simulink model "gps_casestudy_1_4"  (R2023a)
settings: Solver=VariableStepAuto  StartTime=0.0  StopTime=10.0  RelTol=1e-3
settings Model: PacingRate=0.890000  ExtModeTrigDuration=100  Creator=simon  LastModifiedBy=simon
settings DataIOCC: StateSaveName=tmp_raccel_xout  OutputSaveName=tmp_raccel_yout1  SignalLoggingName=tmp_raccel_logsout
settings OptimizationCC: EfficientMapNaN2IntZero=off  AccelVerboseBuild=on
settings HardwareCC: TargetBitPerPointer=64  TargetBitPerSizeT=64  TargetBitPerPtrDiffT=64  TargetLongLongMode=on  TargetIntDivRoundTo=Zero  TargetEndianess=LittleEndian  TargetWordSize=64  TargetHWDeviceType=MATLAB Host  ProdEqTarget=off
settings RTWCC: SystemTargetFile=raccel.tlc  TemplateMakefile=raccel_default_tmf  RTWVerbose=off  RTWUseSimCustomCode=on
settings CodeAppCC: GenerateComments=off  MaxIdLength=128  SimulinkBlockComments=off
settings RaccelTargetCC: TargetLangStandard=C99 (ISO)  OptimizeReductions=off  ENABLE_SLEXEC_SSBRIDGE=1  RTWCAPIParams=on  RTWCAPIRootIO=on

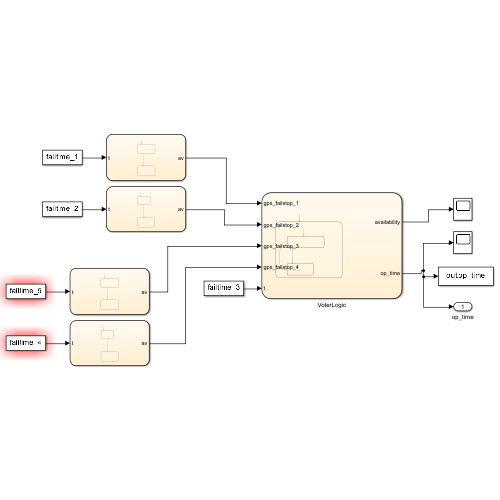
[thumbnail: Simulink's stored preview of the top-level diagram]
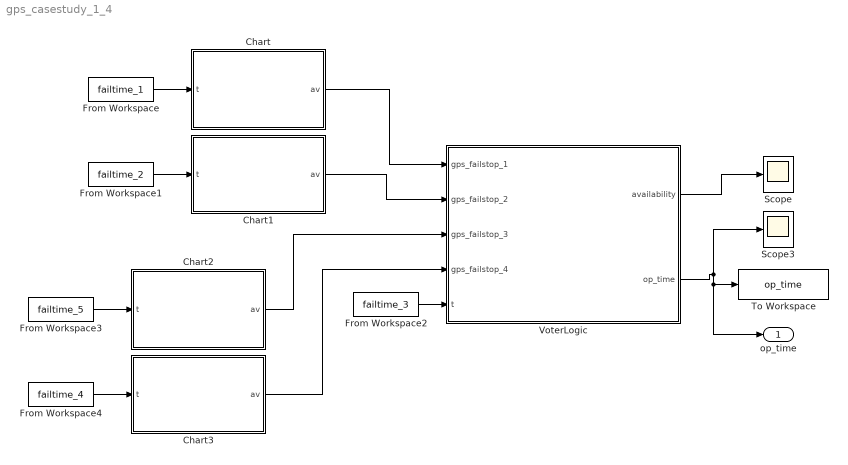
== system gps_casestudy_1_4 ==
  Chart : Stateflow chart  TreatAsAtomicUnit=on
  Chart1 : Stateflow chart  TreatAsAtomicUnit=on
  Chart2 : Stateflow chart  TreatAsAtomicUnit=on
  Chart3 : Stateflow chart  TreatAsAtomicUnit=on
  From Workspace : FromWorkspace  VariableName=failtime_1  SampleTime=-1
  From Workspace1 : FromWorkspace  VariableName=failtime_2  SampleTime=-1
  From Workspace2 : FromWorkspace  VariableName=failtime_3  SampleTime=-1
  From Workspace3 : FromWorkspace  VariableName=failtime_5  SampleTime=-1
  From Workspace4 : FromWorkspace  VariableName=failtime_4  SampleTime=-1
  Scope : Scope
  Scope3 : Scope
  To Workspace : ToWorkspace  VariableName=op_time  SaveFormat=Timeseries  SampleTime=-1
  VoterLogic : Stateflow chart  TreatAsAtomicUnit=on
  op_time : Outport
  wires:
  VoterLogic/1(availability) -> Scope/1
  VoterLogic/2(op_time) -> Scope3/1, To Workspace/1, op_time/1
  From Workspace1/1 -> Chart1/1(t)
  From Workspace/1 -> Chart/1(t)
  Chart/1(av) -> VoterLogic/1(gps_failstop_1)
  Chart1/1(av) -> VoterLogic/2(gps_failstop_2)
  From Workspace2/1 -> VoterLogic/5(t)
  Chart3/1(av) -> VoterLogic/4(gps_failstop_4)
  Chart2/1(av) -> VoterLogic/3(gps_failstop_3)
  From Workspace3/1 -> Chart2/1(t)
  From Workspace4/1 -> Chart3/1(t)

== stateflow chart gps_casestudy_1_4/VoterLogic ==
  settings: updateMethod=CONTINUOUS  sampleTime=0.01  executeAtInitialization=1
  state reg2
    state Operation
      exit:
      op_time=temporalCount(sec)
    state Failstop
      entry: availability=0;
    (default) -> Operation : {availability=1}
    Operation -> Failstop [order 2] : after(t,sec)
    Operation -> Failstop [order 1] : [gps_failstop_1==0 && gps_failstop_2==0 && gps_failstop_3==0 && gps_failstop_4==0]
  (default) -> reg2
  data: availability output; op_time output double; gps_failstop_1 input; gps_failstop_2 input; gps_failstop_3 input; gps_failstop_4 input; t input

== stateflow chart gps_casestudy_1_4/Chart2 ==
  settings: updateMethod=CONTINUOUS
  state operational
    entry:
    av=1
  state failstop
    entry:
    av=0;
  (default) -> operational
  operational -> failstop : after(t,sec)
  data: t input double; av output

== stateflow chart gps_casestudy_1_4/Chart3 ==
  settings: updateMethod=CONTINUOUS
  state operational
    entry:
    av=1;
  state failstop
    entry:
    av=0;
  (default) -> operational
  operational -> failstop : after(t,sec)
  data: t input double; av output

== stateflow chart gps_casestudy_1_4/Chart ==
  settings: updateMethod=CONTINUOUS
  state operational
    entry:
    av=1
  state failstop
    entry:
    av=0;
  (default) -> operational
  operational -> failstop : after(t,sec)
  data: t input double; av output

== stateflow chart gps_casestudy_1_4/Chart1 ==
  settings: updateMethod=CONTINUOUS
  state operational
    entry:
    av=1;
  state failstop
    entry:
    av=0;
  (default) -> operational
  operational -> failstop : after(t,sec)
  data: t input double; av output
